simulink model "THEFINAL"  (R2020b)
settings: Solver=VariableStepAuto  StartTime=0.0  StopTime=60  RelTol=1e-3
values from neighbouring files (symbols this model uses):
  A_2 = zeros(3)    [Trial_Script.m]
  A_AD = horzcat(A_i, A_ii)    [Trial_Script.m]
  A_kal = [0 0 0 1 0 0 ... (first row only)    [Trial_Script.m]
  B_2 = I_inv    [Trial_Script.m]
  B_AD = horzcat(B_i, B_ii)    [Trial_Script.m]
  B_kal = [0 0 0 0 0 0 ... (first row only)    [Trial_Script.m]
  C_2 = eye(3)    [Trial_Script.m]
  C_AD = eye(6)    [Trial_Script.m]
  C_kal = eye(6)    [Trial_Script.m]
  D_2 = zeros(3)    [Trial_Script.m]
  D_AD = zeros(6)    [Trial_Script.m]
  D_kal = zeros(6)    [Trial_Script.m]
  f_prop = 100    [Trial_Script.m]
  Fb1_l = -100000    [Trial_Script.m]
  Fb1_u = 100000    [Trial_Script.m]
  Fb2_l = -100000    [Trial_Script.m]
  Fb2_u = 100000    [Trial_Script.m]
  Fb3_l = -100000    [Trial_Script.m]
  Fb3_u = 100000    [Trial_Script.m]
  Fb4_l = -100000    [Trial_Script.m]
  Fb4_u = 100000    [Trial_Script.m]
  Fc1_l = -30000    [Trial_Script.m]
  Fc1_u = 30000    [Trial_Script.m]
  Fc2_l = -30000    [Trial_Script.m]
  Fc2_u = 30000    [Trial_Script.m]
  Fc3_l = -30000    [Trial_Script.m]
  Fc3_u = 30000    [Trial_Script.m]
  Ft1_l = -100000    [Trial_Script.m]
  Ft1_u = 100000    [Trial_Script.m]
  Ft2_l = -100000    [Trial_Script.m]
  Ft2_u = 100000    [Trial_Script.m]
  Ft3_l = -100000    [Trial_Script.m]
  Ft3_u = 100000    [Trial_Script.m]
  Ft4_l = -100000    [Trial_Script.m]
  Ft4_u = 100000    [Trial_Script.m]
  g = 9.81    [Trial_Script.m]
  m = 645    [Trial_Script.m]    (also in testing_file.m = (abs(max(z)) + abs(min(z)))/(abs(max(y)) + abs(min(y))); wind_stuff.m = (abs(max(z)) + abs(min(z)))/(abs(max(y)) + abs(min(y))))
  r_0 = Tzy_Shard*[90; -125; 160]    [Trial_Script.m]
  rho = 1.225    [Trial_Script.m]
  T = 10.5    [Trial_Script.m]
  time_delay = 0.1    [Trial_Script.m]
  Tx_aero = [1 0 0 ... (first row only)    [Trial_Script.m]
  Tzy_Shard = [cos(pi/2) -sin(pi/2) 0; sin(pi/2) cos(pi/2) 0; 0 0 1]*[1 0 0 ... (first row only)    [Reading_Shard_Data.m]    (also in Trial_Script.m)
  Tzy_Shard_inv = inv(Tzy_Shard)    [Trial_Script.m]
  u_0 = a(1:d,1)    [Reading_Shard_Data.m]    (also in Trial_Script.m = a(1:d_shard,1); testing_file.m)
  u_1 = a(1:d,2)    [Reading_Shard_Data.m]    (also in Trial_Script.m = a(1:d_shard,2); testing_file.m)
  u_2 = a(1:d,3)    [Reading_Shard_Data.m]    (also in Trial_Script.m = a(1:d_shard,3); testing_file.m)
  v_0 = Tzy_Shard*V0_shard    [Trial_Script.m]
  w_0 = [0;0;0]    [Trial_Script.m]
  xdata = a(1:d_shard,4)    [Trial_Script.m]
  ydata = a(1:d_shard,5)    [Trial_Script.m]
  zdata = a(1:d_shard,6)    [Trial_Script.m]
  ZI_Cx = model_Cx(XI_Cx, YI_Cx)    [Trial_Script.m]
  ZI_Cy = model_Cy(XI_Cy, YI_Cy)    [Trial_Script.m]
  ZI_Cz = model_Cz(XI_Cz, YI_Cz)    [Trial_Script.m]
  ZI_p = model_p(XI_p, YI_p)    [Trial_Script.m]
  ZI_q = model_q(XI_q, YI_q)    [Trial_Script.m]
  ZI_r = model_r(XI_r, YI_r)    [Trial_Script.m]
undefined symbols (not defined in the file or in its folder): C_D, Continuous, S, Time
libraries: pid_lib x3, dspsigops x3, fuzblock x3, dspindex x3, ctrlSharedLib x2, simulink x1, mpclib x1, dspmathops x1, cstblocks x1
(part 1 of 2)
settings Model: Creator=Jonathan van Zyl  LastModifiedBy=Jonathan van Zyl

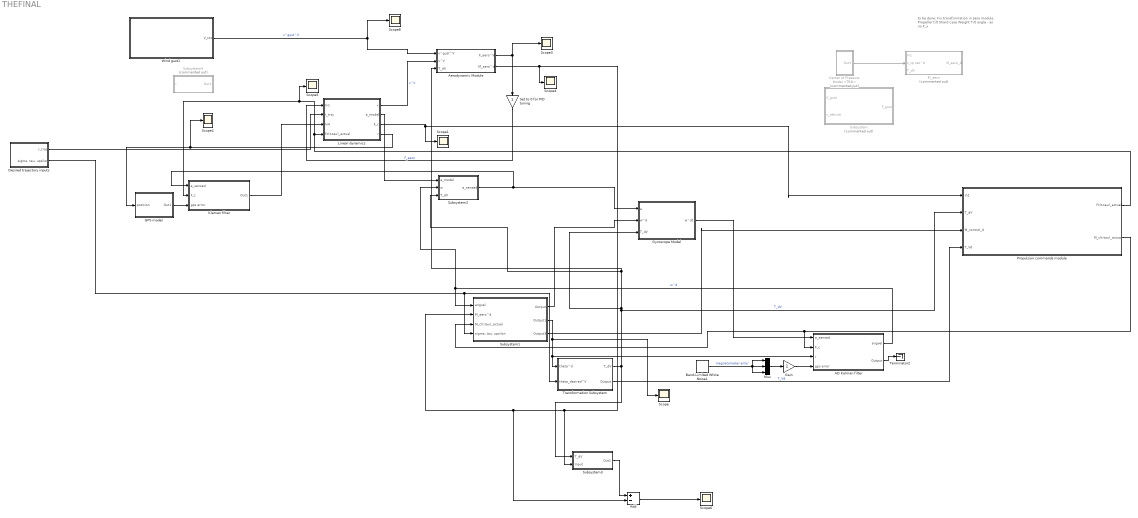
== system THEFINAL ==
  note: to be done:
      | Fix transformation in aero module
      | Propeller tilt
      | Shard case
      | Weight
      | Tilt angle - as no F_x
  AD Kalman filter : Subsystem
  Add : Sum  Inputs=+-
  Aerodynamic Module : Subsystem
  Band-Limited White Noise1 : simulink/Sources/Band-Limited White Noise  Cov=[0.000000001]  Ts=0.1  seed=[23341]
  Center of Pressure Model <TBD> : Subsystem  Commented=on
  Desired trajectory inputs : Subsystem
  GPS model : Subsystem
  Gain : Gain
  Gyroscope Model : Subsystem
  Klaman filter : Subsystem
  Linear dynamics : Subsystem
  M_aero : Subsystem  Commented=on
  Mux : Mux  Inputs=3
  Propulsion commands module : Subsystem
  Scope{,1..6,8} (8 alike) : Scope
  Set to 0 for PID tuning : Gain
  Subsystem : Subsystem  Commented=on
  Subsystem1 : Subsystem
  Subsystem2 : Subsystem
  Subsystem3 : Subsystem
  Subsystem4 : Subsystem  Commented=on
  Terminator2 : Terminator
  Transformation Subsystem : Subsystem
  Wind gust1 : Subsystem
  wires:
  Mux/1 -> Gain/1
  Subsystem3/1(Out1) -> Add/1
  Add/1 -> Scope6/1
  Propulsion commands module/1(Fc(t-tau)_actual) -> Scope5/1, Klaman filter/2(F_c), Linear dynamics/4(Fc(t-tau)_actual)
  Desired trajectory inputs/2("sigma, tau, upsilon") -> Transformation Subsystem/2(theta_desired^V), Subsystem1/4("sigma, tau, upsilon")
  Aerodynamic Module/1(F_aero^V) -> Set to 0 for PID tuning/1, Scope3/1
  Aerodynamic Module/2(M_aero^d) -> Scope4/1, Add/2, Subsystem1/2(M_aero^d), Subsystem3/2(Input)
  Wind gust1/1(V_tot) -> Aerodynamic Module/1(v^gust^V), Scope8/1  "v^gust^V"
  Linear dynamics/1(v) -> Aerodynamic Module/2(v^V)  "v^V"
  Gyroscope Model/1(w^d1) -> AD Kalman filter/1(a_sensed)
  Desired trajectory inputs/1(r_traj) -> Linear dynamics/2(r_traj)
  Propulsion commands module/2(M_c(t-tau)_actual) -> AD Kalman filter/2(F_c), Subsystem1/3(M_c(t-tau)_actual)
  Center of Pressure Model <TBD>/1(Out1) -> M_aero/2(x_cp vec^d)
  Transformation Subsystem/2(Output) -> Propulsion commands module/4(T_Vd)  "T_Vd"
  AD Kalman filter/2(Output) -> Terminator2/1
  Subsystem1/1(Output) -> Gyroscope Model/2(w^d)
  Subsystem1/2(Output1) -> Transformation Subsystem/1(theta^d), AD Kalman filter/3(r), Scope/1
  Subsystem1/3(Output3) -> Propulsion commands module/3(M_control_d)
  AD Kalman filter/1(angvel) -> Subsystem2/2(w), Subsystem1/1(angvel)  "w^d"
  Klaman filter/1(Out1) -> Linear dynamics/3(In4)
  Set to 0 for PID tuning/1 -> Linear dynamics/1(In1)  "F_aero"
  Band-Limited White Noise1/1 -> Mux/1, Mux/2, Mux/3  "magnetometer error"
  GPS model/1(Out1) -> Klaman filter/3(gps error)
  Subsystem2/1(a_sensed) -> Gyroscope Model/1(a), Klaman filter/1(a_sensed)
  Transformation Subsystem/1(T_dV) -> Subsystem3/1(T_dV), Aerodynamic Module/3(T_dV), Subsystem2/3(T_dV), Gyroscope Model/3(T_dV), Propulsion commands module/2(T_dV)  "T_dV"
  Linear dynamics/3(F_c) -> Propulsion commands module/1(In1), Scope1/1
  Gain/1 -> AD Kalman filter/4(gps error)
  Linear dynamics/4(r) -> GPS model/1(position), Scope2/1
  Linear dynamics/2(a_model) -> Subsystem2/1(a_model)

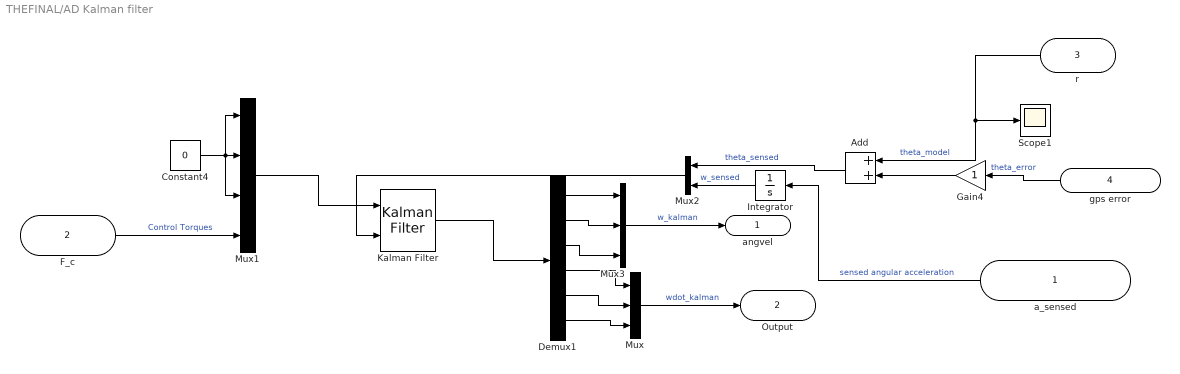
== system THEFINAL/AD Kalman filter ==
  a_sensed : Inport
  F_c : Inport  Port=2
  r : Inport  Port=3
  gps error : Inport  Port=4
  Add : Sum
  Constant4 : Constant  Value=0
  Demux1 : Demux  Outputs=6
  Gain4 : Gain
  Integrator : Integrator  InitialCondition=w_0
  Kalman Filter : ctrlSharedLib/Kalman Filter  TimeDomain=Continuous-Time  UseCurrentEstimator=on  ModelSource=Individual A, B, C, D matrices  ModelSourceVariable=ss(0.95,1,1,0,1)  A=A_AD  B=B_AD  C=C_AD  D=D_AD  NumberOfStates=1  NumberOfInputs=1  NumberOfOutputs=1  InitialEstimateSource=Dialog  X0=[0;0;0;0;0;0]  P0=10  UseK=off  UseGH=off  NumberOfProcessNoiseInputs=1  G=1  TimeInvariantG=on  H=0  TimeInvariantH=on  Q=0.05  TimeInvariantQ=on  R=1  TimeInvariantR=on  N=0  TimeInvariantN=on  AddInputPort=on  AddEnablePort=off  OutputEstimatedY=off  OutputP=off  Ts=-1
  Mux : Mux  Inputs=3
  Mux1 : Mux
  Mux2 : Mux  Inputs=2
  Mux3 : Mux  Inputs=3
  Scope1 : Scope
  angvel : Outport
  Output : Outport  Port=2
  wires:
  Demux1/5 -> Mux/2
  Mux2/1 -> Kalman Filter/2
  Constant4/1 -> Mux1/3, Mux1/1, Mux1/2
  gps error/1 -> Gain4/1  "theta_error"
  r/1 -> Scope1/1, Add/1  "theta_model"
  Demux1/4 -> Mux/1
  Demux1/2 -> Mux3/2
  Mux1/1 -> Kalman Filter/1
  F_c/1 -> Mux1/4  "Control Torques"
  Demux1/1 -> Mux3/1
  Kalman Filter/1 -> Demux1/1
  Demux1/6 -> Mux/3
  Gain4/1 -> Add/2
  Demux1/3 -> Mux3/3
  Integrator/1 -> Mux2/2  "w_sensed"
  Add/1 -> Mux2/1  "theta_sensed"
  Mux3/1 -> angvel/1  "w_kalman"
  a_sensed/1 -> Integrator/1  "sensed angular acceleration"
  Mux/1 -> Output/1  "wdot_kalman"

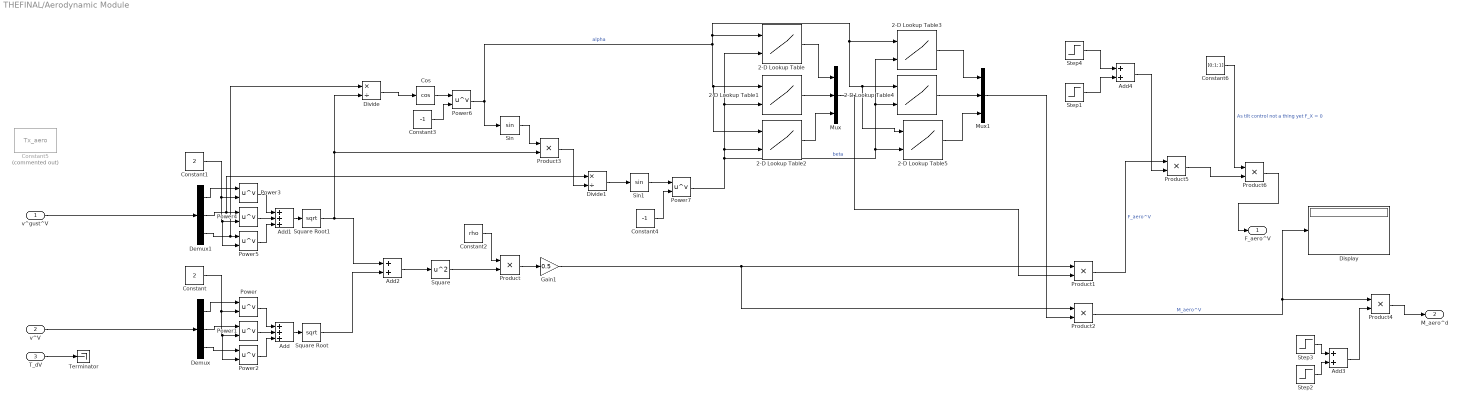
== system THEFINAL/Aerodynamic Module ==
  v^gust^V : Inport
  v^V : Inport  Port=2
  T_dV : Inport  Port=3
  2-D Lookup Table : Lookup_n-D  BreakpointsForDimension1=[-180:1:180]  BreakpointsForDimension2=[-180:1:180]  Table=ZI_Cx  InternalRulePriority=Speed  RndMeth=Simplest  InputSameDT=on
      settings: InputPortMap=u0,u1
  2-D Lookup Table1 : Lookup_n-D  BreakpointsForDimension1=[-180:1:180]  BreakpointsForDimension2=[-180:1:180]  Table=ZI_Cy  InternalRulePriority=Speed  RndMeth=Simplest  InputSameDT=on
      settings: InputPortMap=u0,u1
  2-D Lookup Table2 : Lookup_n-D  BreakpointsForDimension1=[-180:1:180]  BreakpointsForDimension2=[-180:1:180]  Table=ZI_Cz  InternalRulePriority=Speed  RndMeth=Simplest  InputSameDT=on
      settings: InputPortMap=u0,u1
  2-D Lookup Table3 : Lookup_n-D  BreakpointsForDimension1=[-180:1:180]  BreakpointsForDimension2=[-180:1:180]  Table=ZI_p  InternalRulePriority=Speed  RndMeth=Simplest  InputSameDT=on
      settings: InputPortMap=u0,u1
  2-D Lookup Table4 : Lookup_n-D  BreakpointsForDimension1=[-180:1:180]  BreakpointsForDimension2=[-180:1:180]  Table=ZI_q  InternalRulePriority=Speed  RndMeth=Simplest  InputSameDT=on
      settings: InputPortMap=u0,u1
  2-D Lookup Table5 : Lookup_n-D  BreakpointsForDimension1=[-180:1:180]  BreakpointsForDimension2=[-180:1:180]  Table=ZI_r  InternalRulePriority=Speed  RndMeth=Simplest  InputSameDT=on
      settings: InputPortMap=u0,u1
  Add : Sum  Inputs=+++
  Add1 : Sum  Inputs=+++
  Add2 : Sum
  Add3 : Sum
  Add4 : Sum
  Constant : Constant  Value=2
  Constant1 : Constant  Value=2
  Constant2 : Constant  Value=rho
  Constant3 : Constant  Value=-1
  Constant4 : Constant  Value=-1
  Constant5 : Constant  Commented=on  Value=Tx_aero
  Constant6 : Constant  Value=[0;1;1]
  Cos : Trigonometry  Operator=cos
  Demux : Demux  Outputs=3
  Demux1 : Demux  Outputs=3
  Display : Display
  Divide : Product  Inputs=*/
  Divide1 : Product  Inputs=*/
  Gain1 : Gain  Gain=0.5
  Mux : Mux  Inputs=3
  Mux1 : Mux  Inputs=3
  Power{,1..7} (8 alike) : Math  Operator=pow  SaturateOnIntegerOverflow=on
  Product{,1..6} (7 alike) : Product
  Sin : Trigonometry
  Sin1 : Trigonometry
  Square : Math  Operator=square  SaturateOnIntegerOverflow=on
  Square Root : Sqrt  SaturateOnIntegerOverflow=on
  Square Root1 : Sqrt  SaturateOnIntegerOverflow=on
  Step1 : Step  Time=0  SampleTime=0
  Step2 : Step  Time=0  SampleTime=0
  Step3 : Step  Time=10.5  After=-1  SampleTime=0
  Step4 : Step  Time=10.5  After=-1  SampleTime=0
  Terminator : Terminator
  F_aero^V : Outport
  M_aero^d : Outport  Port=2
  wires:
  Constant1/1 -> Power5/2, Power4/2, Power3/2
  Product1/1 -> Product5/1  "F_aero^V"
  Square Root/1 -> Add2/2
  Power6/1 -> Sin/1, 2-D Lookup Table/1, 2-D Lookup Table5/1, 2-D Lookup Table4/1, 2-D Lookup Table3/1, 2-D Lookup Table2/1, 2-D Lookup Table1/1  "alpha"
  Power1/1 -> Add/2
  2-D Lookup Table5/1 -> Mux1/3
  Constant/1 -> Power2/2, Power1/2, Power/2
  Divide/1 -> Cos/1
  Demux/1 -> Power/1
  Power5/1 -> Add1/3
  2-D Lookup Table/1 -> Mux/1
  Divide1/1 -> Sin1/1
  Demux1/1 -> Power3/1
  Add2/1 -> Square/1
  Product2/1 -> Display/1, Product4/1  "M_aero^V"
  Demux/3 -> Power2/1
  Constant4/1 -> Power7/2
  2-D Lookup Table4/1 -> Mux1/2
  Gain1/1 -> Product2/1, Product1/1
  Constant3/1 -> Power6/2
  Power7/1 -> 2-D Lookup Table/2, 2-D Lookup Table1/2, 2-D Lookup Table2/2, 2-D Lookup Table3/2, 2-D Lookup Table4/2, 2-D Lookup Table5/2  "beta"
  Cos/1 -> Power6/1
  Demux1/3 -> Divide/1, Power5/1
  Product/1 -> Gain1/1
  Sin1/1 -> Power7/1
  Power2/1 -> Add/3
  Sin/1 -> Product3/1
  Mux1/1 -> Product2/2
  Demux1/2 -> Divide1/1, Power4/1
  Power4/1 -> Add1/2
  Add/1 -> Square Root/1
  Power/1 -> Add/1
  Square Root1/1 -> Product3/2, Divide/2, Add2/1
  2-D Lookup Table3/1 -> Mux1/1
  2-D Lookup Table1/1 -> Mux/2
  Power3/1 -> Add1/1
  Mux/1 -> Product1/2
  Product3/1 -> Divide1/2
  2-D Lookup Table2/1 -> Mux/3
  Add1/1 -> Square Root1/1
  Constant2/1 -> Product/1
  Demux/2 -> Power1/1
  Add3/1 -> Product4/2
  Step3/1 -> Add3/1
  Step2/1 -> Add3/2
  Product4/1 -> M_aero^d/1
  Step4/1 -> Add4/1
  Step1/1 -> Add4/2
  Square/1 -> Product/2
  Constant6/1 -> Product6/1  "As tilt control not a thing yet F_X = 0"
  Product6/1 -> F_aero^V/1
  T_dV/1 -> Terminator/1
  v^V/1 -> Demux/1
  Product5/1 -> Product6/2
  Add4/1 -> Product5/2
  v^gust^V/1 -> Demux1/1

== system THEFINAL/Center of Pressure Model <TBD> ==
  Constant1 : Constant  Value=[0.1;0.2; 0.05]
  Out1 : Outport
  wires:
  Constant1/1 -> Out1/1  "x_cp"

== system THEFINAL/Desired trajectory inputs ==
  Constant : Constant  Value=Tzy_Shard
  Constant1 : Constant  Value=[90; 174; 240]
  Constant2 : Constant  Value=[0;1;1]
  Constant3 : Constant  Value=[0;10*pi/180;0]
  Matrix Multiply : Product  Multiplication=Matrix(*)
  Product : Product
  r_traj : Outport
  "sigma, tau, upsilon" : Outport  Port=2
  wires:
  Product/1 -> r_traj/1  "r_traj"
  Constant3/1 -> "sigma, tau, upsilon"/1  "sigma, tau, upsilon"
  Constant/1 -> Matrix Multiply/1
  Constant1/1 -> Matrix Multiply/2
  Constant2/1 -> Product/1
  Matrix Multiply/1 -> Product/2  "r_traj"

== system THEFINAL/GPS model ==
  position : Inport
  GPS Model : MATLAB Function  TreatAsAtomicUnit=on
  Transpose : Math  Operator=transpose  SaturateOnIntegerOverflow=on
  Out1 : Outport
  wires:
  GPS Model/1(newposition) -> Transpose/1  "gps error"
  position/1 -> GPS Model/1(position)
  Transpose/1 -> Out1/1  "r_sensed"

== system THEFINAL/Gyroscope Model ==
  a : Inport
  w^d : Inport  Port=2
  T_dV : Inport  Port=3
  Demux : Demux  Outputs=3
  MATLAB Function : MATLAB Function  TreatAsAtomicUnit=on
  Terminator : Terminator
  Transpose : Math  Operator=transpose  SaturateOnIntegerOverflow=on
  Transpose2 : Math  Operator=transpose  SaturateOnIntegerOverflow=on
  w^d1 : Outport
  wires:
  T_dV/1 -> Terminator/1
  Transpose2/1 -> w^d1/1
  MATLAB Function/1(gyroData) -> Transpose2/1
  a/1 -> Transpose/1
  Transpose/1 -> MATLAB Function/4(acc)
  w^d/1 -> Demux/1
  Demux/1 -> MATLAB Function/1(xvel)
  Demux/2 -> MATLAB Function/2(yvel)
  Demux/3 -> MATLAB Function/3(zvel)

== system THEFINAL/Klaman filter ==
  a_sensed : Inport
  F_c : Inport  Port=2
  gps error : Inport  Port=3
  Constant4 : Constant  Value=0
  Demux1 : Demux  Outputs=6
  Integrator : Integrator  InitialCondition=v_0
  Kalman Filter : ctrlSharedLib/Kalman Filter  TimeDomain=Continuous-Time  UseCurrentEstimator=on  ModelSource=Individual A, B, C, D matrices  ModelSourceVariable=ss(0.95,1,1,0,1)  A=A_kal  B=B_kal  C=C_kal  D=D_kal  NumberOfStates=1  NumberOfInputs=1  NumberOfOutputs=1  InitialEstimateSource=Dialog  X0=[0;0;0;0;0;0]  P0=10  UseK=off  UseGH=off  NumberOfProcessNoiseInputs=1  G=1  TimeInvariantG=on  H=0  TimeInvariantH=on  Q=0.05  TimeInvariantQ=on  R=1  TimeInvariantR=on  N=0  TimeInvariantN=on  AddInputPort=on  AddEnablePort=off  OutputEstimatedY=off  OutputP=off  Ts=-1
  Mux1 : Mux
  Mux2 : Mux  Inputs=2
  Mux3 : Mux  Inputs=3
  Terminator : Terminator
  Terminator1 : Terminator
  Terminator2 : Terminator
  Out1 : Outport
  wires:
  Demux1/5 -> Terminator1/1
  Mux2/1 -> Kalman Filter/2
  Constant4/1 -> Mux1/3, Mux1/1, Mux1/2
  Demux1/4 -> Terminator/1
  Demux1/2 -> Mux3/2
  Mux1/1 -> Kalman Filter/1
  F_c/1 -> Mux1/4  "Control Force"
  Demux1/1 -> Mux3/1
  Kalman Filter/1 -> Demux1/1
  Demux1/6 -> Terminator2/1
  Demux1/3 -> Mux3/3
  Integrator/1 -> Mux2/2  "v_sensed"
  gps error/1 -> Mux2/1  "r_sensed"
  Mux3/1 -> Out1/1  "r_kalman"
  a_sensed/1 -> Integrator/1  "sensed acceleration"

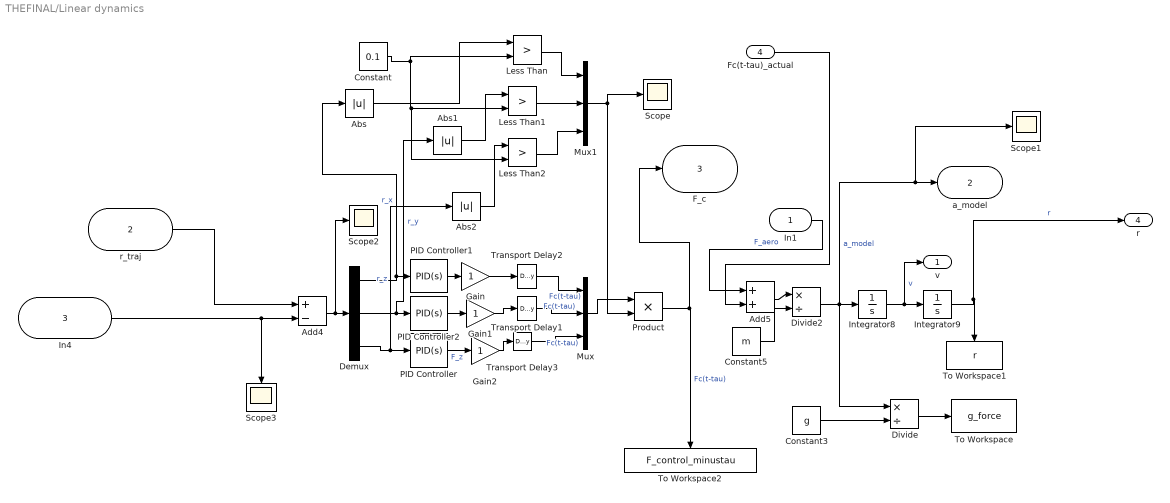
== system THEFINAL/Linear dynamics ==
  In1 : Inport
  r_traj : Inport  Port=2
  In4 : Inport  Port=3
  Fc(t-tau)_actual : Inport  Port=4
  Abs : Abs
  Abs1 : Abs
  Abs2 : Abs
  Add4 : Sum  Inputs=+-
  Add5 : Sum
  Constant : Constant  Value=0.1
  Constant3 : Constant  Value=g
  Constant5 : Constant  Value=m
  Demux : Demux  Outputs=3
  Divide : Product  Inputs=*/
  Divide2 : Product  Inputs=*/
  Gain : Gain
  Gain1 : Gain
  Gain2 : Gain
  Integrator8 : Integrator  InitialCondition=v_0
  Integrator9 : Integrator  InitialCondition=r_0
  Less Than : RelationalOperator  Operator=>  OutDataTypeStr=boolean  RndMeth=Simplest
  Less Than1 : RelationalOperator  Operator=>  OutDataTypeStr=boolean  RndMeth=Simplest
  Less Than2 : RelationalOperator  Operator=>  OutDataTypeStr=boolean  RndMeth=Simplest
  Mux : Mux  Inputs=3
  Mux1 : Mux  Inputs=3
  PID Controller : pid_lib/PID Controller  Controller=PID  Form=Parallel  TimeDomain=Continuous-time  UseExternalTs=off  SampleTime=-1  IntegratorMethod=Forward Euler  FilterMethod=Forward Euler  ControllerParametersSource=internal  P=9009.63914576468  I=3464.3602040453  D=5659.73322598295  UseFilter=on  N=27.0214258529072  TunerSelectOption=Transfer Function Based (PID Tuner App)  InitialConditionSource=internal  InitialConditionForIntegrator=0  InitialConditionForFilter=0  DifferentiatorICPrevScaledInput=0  ExternalReset=none  TrackingMode=off  Kt=1  LimitOutput=off  SatLimitsSource=internal  UpperSaturationLimit=inf  LowerSaturationLimit=-inf  LinearizeAsGain=on  AntiWindupMode=none  Kb=1  POutMin=[]  POutMax=[]  IOutMin=[]  IOutMax=[]  DOutMin=[]  DOutMax=[]  NOutMin=[]  NOutMax=[]  SumOutMin=[]  SumOutMax=[]  SaturationOutMin=[]  SaturationOutMax=[]  PParamMin=[]  PParamMax=[]  IParamMin=[]  IParamMax=[]  DParamMin=[]  DParamMax=[]  NParamMin=[]  NParamMax=[]  KbParamMin=[]  KbParamMax=[]  KtParamMin=[]  KtParamMax=[]  KbOutMin=[]  KbOutMax=[]  KtOutMin=[]  KtOutMax=[]  IntegratorOutMin=[]  IntegratorOutMax=[]  FilterOutMin=[]  FilterOutMax=[]  SumI1OutMin=[]  SumI1OutMax=[]  SumI2OutMin=[]  SumI2OutMax=[]  SumI3OutMin=[]  SumI3OutMax=[]  SumI4OutMin=[]  SumI4OutMax=[]  SumDOutMin=[]  SumDOutMax=[]  DifferentiatorOutMin=[]  DifferentiatorOutMax=[]  FilterDiffOutCoefMin=[]  FilterDiffOutCoefMax=[]  ReciprocalOutMin=[]  ReciprocalOutMax=[]  SumDenOutMin=[]  SumDenOutMax=[]  SumNumOutMin=[]  SumNumOutMax=[]  DivideOutMin=[]  DivideOutMax=[]  UdiffTsProdOutMin=[]  UdiffTsProdOutMax=[]  NTsProdOutMin=[]  NTsProdOutMax=[]  UintegralTsProdOutMin=[]  UintegralTsProdOutMax=[]  UngainTsProdOutMin=[]  UngainTsProdOutMax=[]  IntegratorContinuousStateAttributes=''  IntegratorStateMustResolveToSignalObject=off  IntegratorRTWStateStorageClass=Auto  FilterContinuousStateAttributes=''  FilterStateMustResolveToSignalObject=off  FilterRTWStateStorageClass=Auto  ParallelPVariant=InternalParameters  IdealPVariant=Disabled  IVariant=InternalParameters  DVariant=InternalParameters  IntegratorVariant=Continuous  SatVariant=Disabled  AWVariant=Passthrough  PCopyVariant=Disabled  TRVariant=Disabled  FdbkBlocksVariant=Forward  IdealPFdbkVariant=Disabled  SatFdbkVariant=Disabled  DerivativeFilterVariant=ContFilter  NVariant=InternalParameters  NCopyVariant=Disabled  FilterICVariant=InternalICsFilter  IntegratorICVariant=InternalICs  ExternalResetVariant=Disabled  TRSumVariant=Passthrough  SumFdbkVariant=Disabled  SumVariant=Sum_PID  TsampFilterVariant=InternalTs  TsampNgainVariant=Passthrough  TsampIntegralVariant=Passthrough  ExternalSaturationOutDataTypeStr=Inherit: Same as second input
  PID Controller1 : pid_lib/PID Controller  Controller=PID  Form=Parallel  TimeDomain=Continuous-time  UseExternalTs=off  SampleTime=-1  IntegratorMethod=Forward Euler  FilterMethod=Forward Euler  ControllerParametersSource=internal  P=9009.63914576468  I=3464.36020404063  D=5659.73322596604  UseFilter=on  N=27.0214258528983  TunerSelectOption=Transfer Function Based (PID Tuner App)  InitialConditionSource=internal  InitialConditionForIntegrator=0  InitialConditionForFilter=0  DifferentiatorICPrevScaledInput=0  ExternalReset=none  TrackingMode=off  Kt=1  LimitOutput=off  SatLimitsSource=internal  UpperSaturationLimit=inf  LowerSaturationLimit=-inf  LinearizeAsGain=on  AntiWindupMode=none  Kb=1  POutMin=[]  POutMax=[]  IOutMin=[]  IOutMax=[]  DOutMin=[]  DOutMax=[]  NOutMin=[]  NOutMax=[]  SumOutMin=[]  SumOutMax=[]  SaturationOutMin=[]  SaturationOutMax=[]  PParamMin=[]  PParamMax=[]  IParamMin=[]  IParamMax=[]  DParamMin=[]  DParamMax=[]  NParamMin=[]  NParamMax=[]  KbParamMin=[]  KbParamMax=[]  KtParamMin=[]  KtParamMax=[]  KbOutMin=[]  KbOutMax=[]  KtOutMin=[]  KtOutMax=[]  IntegratorOutMin=[]  IntegratorOutMax=[]  FilterOutMin=[]  FilterOutMax=[]  SumI1OutMin=[]  SumI1OutMax=[]  SumI2OutMin=[]  SumI2OutMax=[]  SumI3OutMin=[]  SumI3OutMax=[]  SumI4OutMin=[]  SumI4OutMax=[]  SumDOutMin=[]  SumDOutMax=[]  DifferentiatorOutMin=[]  DifferentiatorOutMax=[]  FilterDiffOutCoefMin=[]  FilterDiffOutCoefMax=[]  ReciprocalOutMin=[]  ReciprocalOutMax=[]  SumDenOutMin=[]  SumDenOutMax=[]  SumNumOutMin=[]  SumNumOutMax=[]  DivideOutMin=[]  DivideOutMax=[]  UdiffTsProdOutMin=[]  UdiffTsProdOutMax=[]  NTsProdOutMin=[]  NTsProdOutMax=[]  UintegralTsProdOutMin=[]  UintegralTsProdOutMax=[]  UngainTsProdOutMin=[]  UngainTsProdOutMax=[]  IntegratorContinuousStateAttributes=''  IntegratorStateMustResolveToSignalObject=off  IntegratorRTWStateStorageClass=Auto  FilterContinuousStateAttributes=''  FilterStateMustResolveToSignalObject=off  FilterRTWStateStorageClass=Auto  ParallelPVariant=InternalParameters  IdealPVariant=Disabled  IVariant=InternalParameters  DVariant=InternalParameters  IntegratorVariant=Continuous  SatVariant=Disabled  AWVariant=Passthrough  PCopyVariant=Disabled  TRVariant=Disabled  FdbkBlocksVariant=Forward  IdealPFdbkVariant=Disabled  SatFdbkVariant=Disabled  DerivativeFilterVariant=ContFilter  NVariant=InternalParameters  NCopyVariant=Disabled  FilterICVariant=InternalICsFilter  IntegratorICVariant=InternalICs  ExternalResetVariant=Disabled  TRSumVariant=Passthrough  SumFdbkVariant=Disabled  SumVariant=Sum_PID  TsampFilterVariant=InternalTs  TsampNgainVariant=Passthrough  TsampIntegralVariant=Passthrough  ExternalSaturationOutDataTypeStr=Inherit: Same as second input
  PID Controller2 : pid_lib/PID Controller  Controller=PID  Form=Parallel  TimeDomain=Continuous-time  UseExternalTs=off  SampleTime=-1  IntegratorMethod=Forward Euler  FilterMethod=Forward Euler  ControllerParametersSource=internal  P=9009.63914576468  I=3464.36020397681  D=5659.73322587286  UseFilter=on  N=27.0214258527793  TunerSelectOption=Transfer Function Based (PID Tuner App)  InitialConditionSource=internal  InitialConditionForIntegrator=0  InitialConditionForFilter=0  DifferentiatorICPrevScaledInput=0  ExternalReset=none  TrackingMode=off  Kt=1  LimitOutput=off  SatLimitsSource=internal  UpperSaturationLimit=inf  LowerSaturationLimit=-inf  LinearizeAsGain=on  AntiWindupMode=none  Kb=1  POutMin=[]  POutMax=[]  IOutMin=[]  IOutMax=[]  DOutMin=[]  DOutMax=[]  NOutMin=[]  NOutMax=[]  SumOutMin=[]  SumOutMax=[]  SaturationOutMin=[]  SaturationOutMax=[]  PParamMin=[]  PParamMax=[]  IParamMin=[]  IParamMax=[]  DParamMin=[]  DParamMax=[]  NParamMin=[]  NParamMax=[]  KbParamMin=[]  KbParamMax=[]  KtParamMin=[]  KtParamMax=[]  KbOutMin=[]  KbOutMax=[]  KtOutMin=[]  KtOutMax=[]  IntegratorOutMin=[]  IntegratorOutMax=[]  FilterOutMin=[]  FilterOutMax=[]  SumI1OutMin=[]  SumI1OutMax=[]  SumI2OutMin=[]  SumI2OutMax=[]  SumI3OutMin=[]  SumI3OutMax=[]  SumI4OutMin=[]  SumI4OutMax=[]  SumDOutMin=[]  SumDOutMax=[]  DifferentiatorOutMin=[]  DifferentiatorOutMax=[]  FilterDiffOutCoefMin=[]  FilterDiffOutCoefMax=[]  ReciprocalOutMin=[]  ReciprocalOutMax=[]  SumDenOutMin=[]  SumDenOutMax=[]  SumNumOutMin=[]  SumNumOutMax=[]  DivideOutMin=[]  DivideOutMax=[]  UdiffTsProdOutMin=[]  UdiffTsProdOutMax=[]  NTsProdOutMin=[]  NTsProdOutMax=[]  UintegralTsProdOutMin=[]  UintegralTsProdOutMax=[]  UngainTsProdOutMin=[]  UngainTsProdOutMax=[]  IntegratorContinuousStateAttributes=''  IntegratorStateMustResolveToSignalObject=off  IntegratorRTWStateStorageClass=Auto  FilterContinuousStateAttributes=''  FilterStateMustResolveToSignalObject=off  FilterRTWStateStorageClass=Auto  ParallelPVariant=InternalParameters  IdealPVariant=Disabled  IVariant=InternalParameters  DVariant=InternalParameters  IntegratorVariant=Continuous  SatVariant=Disabled  AWVariant=Passthrough  PCopyVariant=Disabled  TRVariant=Disabled  FdbkBlocksVariant=Forward  IdealPFdbkVariant=Disabled  SatFdbkVariant=Disabled  DerivativeFilterVariant=ContFilter  NVariant=InternalParameters  NCopyVariant=Disabled  FilterICVariant=InternalICsFilter  IntegratorICVariant=InternalICs  ExternalResetVariant=Disabled  TRSumVariant=Passthrough  SumFdbkVariant=Disabled  SumVariant=Sum_PID  TsampFilterVariant=InternalTs  TsampNgainVariant=Passthrough  TsampIntegralVariant=Passthrough  ExternalSaturationOutDataTypeStr=Inherit: Same as second input
  Product : Product
  Scope{,1..3} (4 alike) : Scope
  To Workspace : ToWorkspace  VariableName=g_force  SaveFormat=Timeseries  SampleTime=-1
      settings: Save2DSignal=2-D array (concatenate along first dimension)
  To Workspace1 : ToWorkspace  VariableName=r  SaveFormat=Timeseries  SampleTime=-1
  To Workspace2 : ToWorkspace  VariableName=F_control_minustau  SaveFormat=Timeseries  SampleTime=-1
  Transport Delay1 : TransportDelay  DelayTime=time_delay  TransDelayFeedthrough=on
  Transport Delay2 : TransportDelay  DelayTime=time_delay  TransDelayFeedthrough=on
  Transport Delay3 : TransportDelay  DelayTime=time_delay  TransDelayFeedthrough=on
  v : Outport
  a_model : Outport  Port=2
  F_c : Outport  Port=3
  r : Outport  Port=4
  wires:
  Divide2/1 -> Divide/1, Scope1/1, a_model/1, Integrator8/1  "a_model"
  In4/1 -> Add4/2, Scope3/1
  Divide/1 -> To Workspace/1
  r_traj/1 -> Add4/1
  PID Controller2/1 -> Gain1/1
  Add5/1 -> Divide2/1
  Constant5/1 -> Divide2/2
  Demux/1 -> Abs/1, PID Controller1/1  "r_x"
  PID Controller/1 -> Gain2/1  "F_z"
  Gain1/1 -> Transport Delay1/1
  Add4/1 -> Scope2/1, Demux/1
  Integrator9/1 -> r/1, To Workspace1/1  "r"
  Demux/2 -> Abs1/1, PID Controller2/1  "r_y"
  Product/1 -> F_c/1, To Workspace2/1  "Fc(t-tau)"
  PID Controller1/1 -> Gain/1
  Constant3/1 -> Divide/2
  Gain/1 -> Transport Delay2/1
  Demux/3 -> Abs2/1, PID Controller/1  "r_z"
  Gain2/1 -> Transport Delay3/1
  Integrator8/1 -> Integrator9/1, v/1  "v"
  In1/1 -> Add5/1  "F_aero"
  Transport Delay2/1 -> Mux/1  "Fc(t-tau)"
  Transport Delay1/1 -> Mux/2  "Fc(t-tau)"
  Transport Delay3/1 -> Mux/3  "Fc(t-tau)"
  Constant/1 -> Less Than2/2, Less Than1/2, Less Than/2
  Less Than1/1 -> Mux1/2
  Less Than/1 -> Mux1/1
  Less Than2/1 -> Mux1/3
  Mux/1 -> Product/1
  Abs/1 -> Less Than/1
  Abs1/1 -> Less Than1/1
  Abs2/1 -> Less Than2/1
  Fc(t-tau)_actual/1 -> Add5/2
  Mux1/1 -> Product/2, Scope/1

== system THEFINAL/M_aero ==
  In1 : Inport
  x_cp vec^d : Inport  Port=2
  T_dV : Inport  Port=3
  Matrix Multiply : Product  Multiplication=Matrix(*)
  Matrix Multiply1 : Product
  M_aero_d : Outport
  wires:
  Matrix Multiply/1 -> Matrix Multiply1/2  "F_dis^d"
  x_cp vec^d/1 -> Matrix Multiply1/1  "x_cp"
  T_dV/1 -> Matrix Multiply/1
  In1/1 -> Matrix Multiply/2  "F_gust"
  Matrix Multiply1/1 -> M_aero_d/1  "M_aero_d"

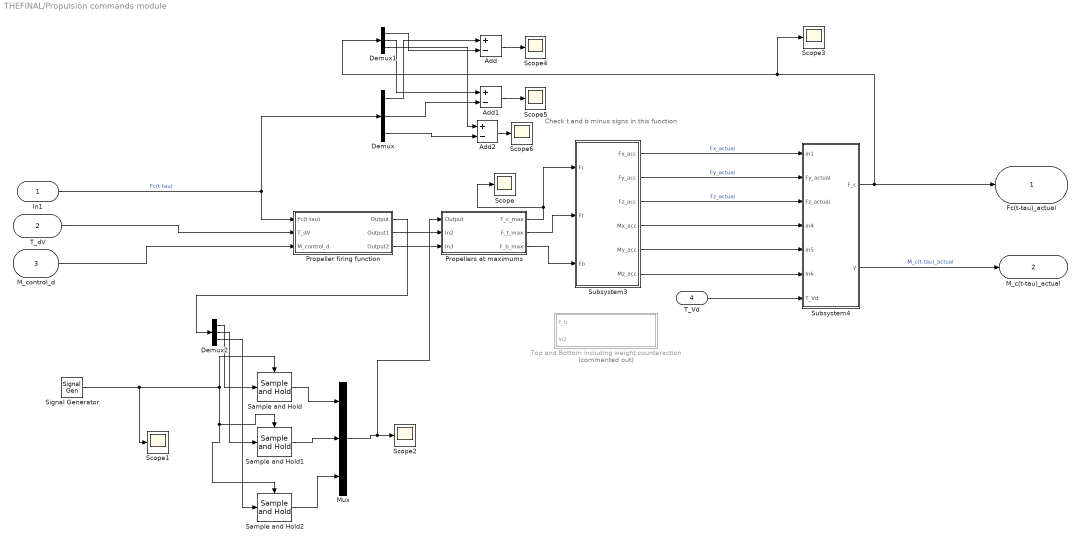
== system THEFINAL/Propulsion commands module ==
  note: Check t and b minus signs in this function
  In1 : Inport
  T_dV : Inport  Port=2
  M_control_d : Inport  Port=3
  T_Vd : Inport  Port=4
  Add : Sum  Inputs=+-
  Add1 : Sum  Inputs=+-
  Add2 : Sum  Inputs=+-
  Demux : Demux  Outputs=3
  Demux1 : Demux  Outputs=3
  Demux2 : Demux  Outputs=3
  Mux : Mux  Inputs=3
  Propeller firing function : Subsystem
  Propellers at maximums : Subsystem
  Sample and Hold : dspsigops/Sample and Hold  trig=Either edge  initCond=0  latchinput=off
  Sample and Hold1 : dspsigops/Sample and Hold  trig=Either edge  initCond=0  latchinput=off
  Sample and Hold2 : dspsigops/Sample and Hold  trig=Either edge  initCond=0  latchinput=off
  Scope{,1..6} (7 alike) : Scope
  Signal Generator : SignalGenerator  WaveForm=square  Frequency=f_prop  Units=rad/sec
  Subsystem3 : Subsystem
  Subsystem4 : Subsystem
  Top and Bottom including weight counteraction : Subsystem  Commented=on
  Fc(t-tau)_actual : Outport
  M_c(t-tau)_actual : Outport  Port=2
  wires:
  Subsystem3/2(Fy_acc) -> Subsystem4/2(Fy_actual)  "Fy_actual"
  Subsystem4/1(F_c) -> Fc(t-tau)_actual/1, Scope3/1, Demux1/1
  Demux1/3 -> Add2/1
  Subsystem3/3(Fz_acc) -> Subsystem4/3(Fz_actual)  "Fz_actual"
  Demux/2 -> Add1/2
  T_dV/1 -> Propeller firing function/2(T_dV)
  Subsystem3/1(Fx_acc) -> Subsystem4/1(In1)  "Fx_actual"
  Demux1/2 -> Add1/1
  Propeller firing function/1(Output) -> Demux2/1
  Propellers at maximums/2(F_t_max) -> Subsystem3/2(Ft)
  Demux1/1 -> Add/2
  Propeller firing function/2(Output1) -> Propellers at maximums/2(In2)
  Subsystem3/5(My_acc) -> Subsystem4/5(In5)
  Subsystem3/6(Mz_acc) -> Subsystem4/6(In6)
  Propellers at maximums/3(F_b_max) -> Subsystem3/3(Fb)
  Demux/3 -> Add2/2
  Subsystem4/2(y) -> M_c(t-tau)_actual/1  "M_c(t-tau)_actual"
  Propeller firing function/3(Output2) -> Propellers at maximums/3(In3)
  In1/1 -> Demux/1, Propeller firing function/1(Fc(t-tau))  "Fc(t-tau)"
  T_Vd/1 -> Subsystem4/7(T_Vd)
  Subsystem3/4(Mx_acc) -> Subsystem4/4(In4)
  Add1/1 -> Scope5/1
  Propellers at maximums/1(F_c_max) -> Scope/1, Subsystem3/1(Fc)
  Add2/1 -> Scope6/1
  Demux/1 -> Add/1
  Add/1 -> Scope4/1
  M_control_d/1 -> Propeller firing function/3(M_control_d)
  Sample and Hold/1 -> Mux/1
  Signal Generator/1 -> Scope1/1, Sample and Hold/Trigger, Sample and Hold2/Trigger, Sample and Hold1/Trigger
  Demux2/1 -> Sample and Hold/1
  Demux2/2 -> Sample and Hold1/1
  Sample and Hold1/1 -> Mux/2
  Sample and Hold2/1 -> Mux/3
  Mux/1 -> Propellers at maximums/1(Output), Scope2/1
  Demux2/3 -> Sample and Hold2/1

== system THEFINAL/Subsystem ==
  V_gust : Inport
  v_vehicle : Inport  Port=2
  Add2 : Sum
  Add3 : Sum
  Drag1 : Subsystem
  Product : Product
  Scope : Scope
  Step2 : Step  Time=0  SampleTime=0
  Step3 : Step  Time=10.5  After=-1  SampleTime=0
  To Workspace : ToWorkspace  VariableName=v_sumsq  SampleTime=-1
  To Workspace1 : ToWorkspace  VariableName=step  SaveFormat=Timeseries  SampleTime=-1
  To Workspace2 : ToWorkspace  VariableName=vtotal  SaveFormat=Timeseries  SampleTime=-1
  To Workspace3 : ToWorkspace  VariableName=F_gust  SaveFormat=Timeseries  SampleTime=-1
  To Workspace4 : ToWorkspace  VariableName=v_gust  SaveFormat=Timeseries  SampleTime=-1
  F_gust : Outport
  wires:
  Product/1 -> F_gust/1, To Workspace3/1, Scope/1  "F_gust"
  Step3/1 -> Add2/1
  V_gust/1 -> To Workspace4/1, Add3/1
  Drag1/1(Out1) -> To Workspace/1
  Add3/1 -> Drag1/1(In1), To Workspace2/1
  Add2/1 -> To Workspace1/1, Product/2
  Step2/1 -> Add2/2
  v_vehicle/1 -> Add3/2
  Drag1/2(drag) -> Product/1

== system THEFINAL/Subsystem1 ==
  angvel : Inport
  M_aero^d : Inport  Port=2
  M_c(t-tau)_actual : Inport  Port=3
  "sigma, tau, upsilon" : Inport  Port=4
  Subsystem : Subsystem
  Output : Outport
  Output1 : Outport  Port=2
  Output3 : Outport  Port=3
  wires:
  M_aero^d/1 -> Subsystem/1(M_aero^d)  "M_aero^d"
  "sigma, tau, upsilon"/1 -> Subsystem/2(Input)  "sigma, tau upsilon"
  Subsystem/1(Output) -> Output1/1  "theta^d"
  Subsystem/2(Output1) -> Output3/1
  Subsystem/3(Out1) -> Output/1
  angvel/1 -> Subsystem/3(angvel)  "angelvel"
  M_c(t-tau)_actual/1 -> Subsystem/4(M_c(t-tau)_actual)

== system THEFINAL/Subsystem2 ==
  a_model : Inport
  w : Inport  Port=2
  T_dV : Inport  Port=3
  Display : Display
  Display1 : Display
  MATLAB Function : MATLAB Function  Commented=on  TreatAsAtomicUnit=on
  Terminator : Terminator
  Terminator3 : Terminator
  Transpose : Math  Operator=transpose  SaturateOnIntegerOverflow=on
  Transpose1 : Math  Operator=transpose  SaturateOnIntegerOverflow=on
  Transpose2 : Math  Operator=transpose  SaturateOnIntegerOverflow=on
  a_sensed : Outport
  wires:
  T_dV/1 -> Terminator3/1
  a_model/1 -> Transpose1/1
  Transpose2/1 -> a_sensed/1  "a_sensed"
  w/1 -> Transpose/1
  Transpose/1 -> Terminator/1
  Transpose1/1 -> Display1/1, Transpose2/1, Display/1  "a_sensed"

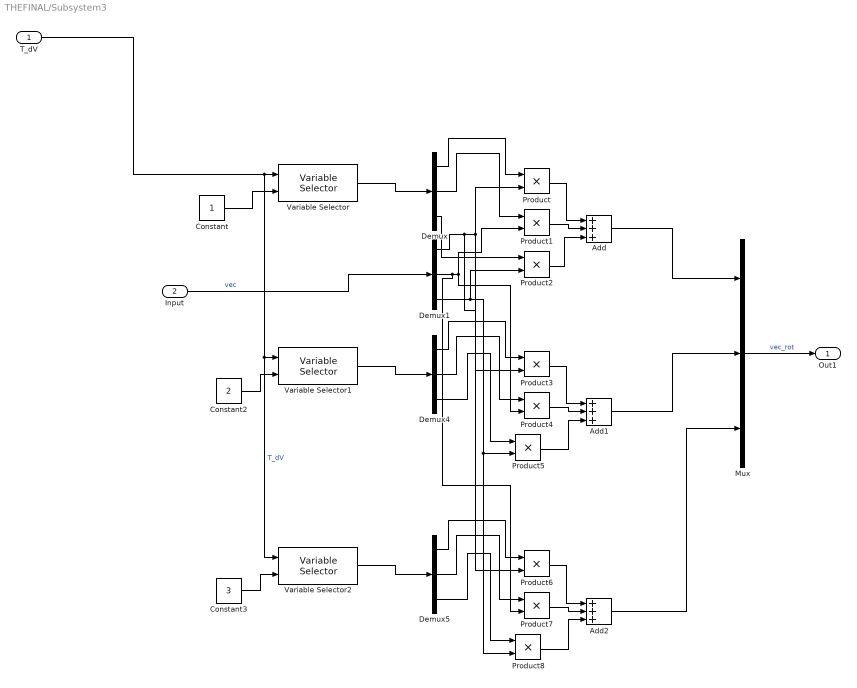
== system THEFINAL/Subsystem3 ==
  T_dV : Inport
  Input : Inport  Port=2
  Add : Sum  Inputs=+++
  Add1 : Sum  Inputs=+++
  Add2 : Sum  Inputs=+++
  Constant : Constant
  Constant2 : Constant  Value=2
  Constant3 : Constant  Value=3
  Demux{,1,4..5} (4 alike) : Demux  Outputs=3
  Mux : Mux  Inputs=3
  Product{,1..8} (9 alike) : Product
  Variable Selector : dspindex/Variable Selector  NumInputs=1  rowsOrCols=Columns  IdxMode=Variable  Elements=[1 3]  ZerOneIdxMode=One-based  errmode=Clip Index  FillMode=on  FillValues=0
  Variable Selector1 : dspindex/Variable Selector  NumInputs=1  rowsOrCols=Columns  IdxMode=Variable  Elements=[1 3]  ZerOneIdxMode=One-based  errmode=Clip Index  FillMode=on  FillValues=0
  Variable Selector2 : dspindex/Variable Selector  NumInputs=1  rowsOrCols=Columns  IdxMode=Variable  Elements=[1 3]  ZerOneIdxMode=One-based  errmode=Clip Index  FillMode=on  FillValues=0
  Out1 : Outport
  wires:
  Variable Selector/1 -> Demux/1
  Add2/1 -> Mux/3
  Demux/1 -> Product/1
  Product3/1 -> Add1/1
  Variable Selector1/1 -> Demux4/1
  Product4/1 -> Add1/2
  Demux4/2 -> Product4/1
  Demux/2 -> Product1/1
  Constant2/1 -> Variable Selector1/2
  Constant/1 -> Variable Selector/2
  Mux/1 -> Out1/1  "vec_rot"
  Add/1 -> Mux/1
  Product5/1 -> Add1/3
  Demux1/2 -> Product7/2, Product1/2, Product4/2
  Product/1 -> Add/1
  Demux5/2 -> Product7/1
  Product8/1 -> Add2/3
  Demux5/3 -> Product8/1
  Product7/1 -> Add2/2
  Demux5/1 -> Product6/1
  Product6/1 -> Add2/1
  Constant3/1 -> Variable Selector2/2
  Demux/3 -> Product2/1
  Variable Selector2/1 -> Demux5/1
  Demux1/3 -> Product8/2, Product5/2, Product2/2
  Product2/1 -> Add/3
  Add1/1 -> Mux/2
  Product1/1 -> Add/2
  Demux4/1 -> Product3/1
  Demux4/3 -> Product5/1
  T_dV/1 -> Variable Selector2/1, Variable Selector1/1, Variable Selector/1  "T_dV"
  Demux1/1 -> Product6/2, Product/2, Product3/2
  Input/1 -> Demux1/1  "vec"

== system THEFINAL/Subsystem4 ==
  r : Inport
  Constant : Constant  Value=xdata
  Constant1 : Constant  Value=ydata
  Constant2 : Constant  Value=zdata
  Constant3 : Constant  Value=Tzy_Shard_inv
  Constant4 : Constant  Value=Tzy_Shard
  Constant5 : Constant  Value=u_0
  Constant6 : Constant  Value=u_1
  Constant7 : Constant  Value=u_2
  Demux : Demux  Outputs=3
  MATLAB Function : MATLAB Function  TreatAsAtomicUnit=on
  Matrix Multiply : Product  Multiplication=Matrix(*)
  Matrix Multiply1 : Product  Multiplication=Matrix(*)
  Mux : Mux  Inputs=3
  Out1 : Outport
  wires:
  Demux/1 -> MATLAB Function/7(xpos)
  Demux/2 -> MATLAB Function/8(ypos)
  Demux/3 -> MATLAB Function/9(zpos)
  r/1 -> Matrix Multiply/2  "r^V"
  Constant/1 -> MATLAB Function/4(xdata)
  Constant1/1 -> MATLAB Function/5(ydata)
  Constant2/1 -> MATLAB Function/6(zdata)
  MATLAB Function/1(u0) -> Mux/1
  MATLAB Function/2(u1) -> Mux/2
  Constant3/1 -> Matrix Multiply/1
  Matrix Multiply/1 -> Demux/1
  Constant4/1 -> Matrix Multiply1/1
  Mux/1 -> Matrix Multiply1/2
  Matrix Multiply1/1 -> Out1/1  "v_gust^V"
  MATLAB Function/3(u2) -> Mux/3
  Constant5/1 -> MATLAB Function/1(u_0)
  Constant6/1 -> MATLAB Function/2(u_1)
  Constant7/1 -> MATLAB Function/3(u_2)

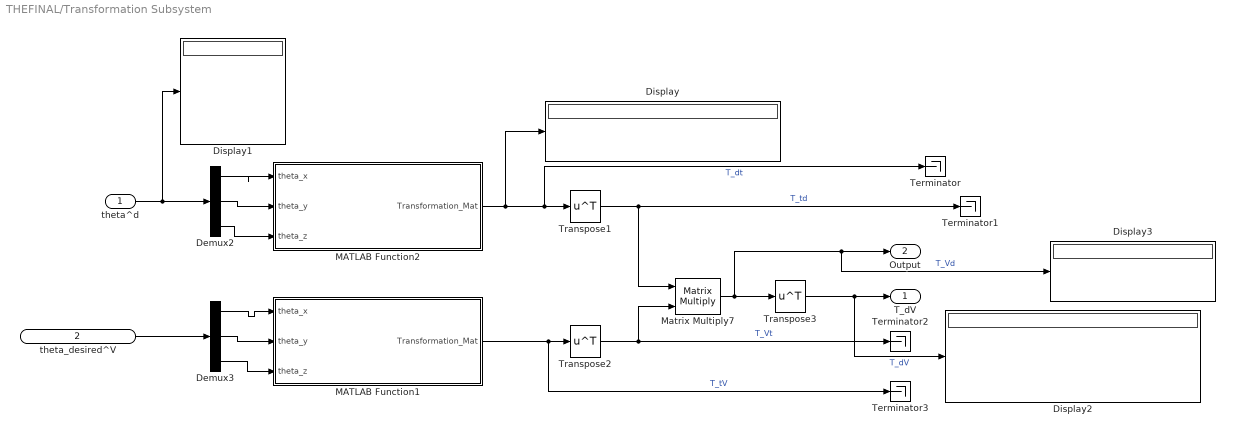
== system THEFINAL/Transformation Subsystem ==
  theta^d : Inport
  theta_desired^V : Inport  Port=2
  Demux2 : Demux  Outputs=3
  Demux3 : Demux  Outputs=3
  Display{,1..3} (4 alike) : Display
  MATLAB Function1 : MATLAB Function  TreatAsAtomicUnit=on
  MATLAB Function2 : MATLAB Function  TreatAsAtomicUnit=on
  Matrix Multiply7 : Product  Multiplication=Matrix(*)
  Terminator{,1..3} (4 alike) : Terminator
  Transpose1 : Math  Operator=transpose  SaturateOnIntegerOverflow=on
  Transpose2 : Math  Operator=transpose  SaturateOnIntegerOverflow=on
  Transpose3 : Math  Operator=transpose  SaturateOnIntegerOverflow=on
  T_dV : Outport
  Output : Outport  Port=2
  wires:
  Demux3/1 -> MATLAB Function1/1(theta_x)
  Demux2/1 -> MATLAB Function2/1(theta_x)
  Transpose2/1 -> Terminator2/1, Matrix Multiply7/2  "T_Vt"
  Demux2/2 -> MATLAB Function2/2(theta_y)
  MATLAB Function2/1(Transformation_Mat) -> Display/1, Terminator/1, Transpose1/1  "T_dt"
  Transpose1/1 -> Terminator1/1, Matrix Multiply7/1  "T_td"
  Demux2/3 -> MATLAB Function2/3(theta_z)
  MATLAB Function1/1(Transformation_Mat) -> Terminator3/1, Transpose2/1  "T_tV"
  Matrix Multiply7/1 -> Display3/1, Output/1, Transpose3/1  "T_Vd"
  theta_desired^V/1 -> Demux3/1
  Demux3/3 -> MATLAB Function1/3(theta_z)
  Demux3/2 -> MATLAB Function1/2(theta_y)
  theta^d/1 -> Display1/1, Demux2/1
  Transpose3/1 -> Display2/1, T_dV/1  "T_dV"

== system THEFINAL/Wind gust1 ==
  Add : Sum  Inputs=+-
  Add1 : Sum  Inputs=+-
  Constant : Constant  Value=12.4
  Constant1 : Constant  Value=4.25
  Constant2 : Constant
  Constant3 : Constant  Value=0
  Constant4 : Constant  Value=0  VectorParams1D=off
  Mux : Mux  Inputs=3
  Product : Product
  Product1 : Product
  Sine Wave : Sin  Frequency=3*pi/T  SampleTime=0
  Sine Wave1 : Sin  Frequency=2*pi/T  Phase=pi/2  SampleTime=0
  V_tot : Outport
  wires:
  Constant/1 -> Add/1
  Constant1/1 -> Product/1
  Sine Wave/1 -> Product/2
  Constant2/1 -> Add1/1
  Sine Wave1/1 -> Add1/2
  Product/1 -> Product1/1
  Add1/1 -> Product1/2
  Product1/1 -> Add/2
  Add/1 -> Mux/2  "v_gust_y"
  Constant3/1 -> Mux/3  "v_gust_z"
  Constant4/1 -> Mux/1  "v_gust_x"
  Mux/1 -> V_tot/1

== system THEFINAL/Propulsion commands module/Propeller firing function ==
  Fc(t-tau) : Inport
  T_dV : Inport  Port=2
  M_control_d : Inport  Port=3
  Gain6 : Gain
  MATLAB Function : MATLAB Function  TreatAsAtomicUnit=on
  Matrix Multiply5 : Product  Multiplication=Matrix(*)
  To Workspace : ToWorkspace  VariableName=Fc_wanted  SaveFormat=Timeseries  SampleTime=-1
  To Workspace1 : ToWorkspace  VariableName=Ft_wanted  SaveFormat=Timeseries  SampleTime=-1
  To Workspace2 : ToWorkspace  VariableName=Fb_wanted  SaveFormat=Timeseries  SampleTime=-1
  Turn off for PID tune : Gain
  Output : Outport
  Output1 : Outport  Port=2
  Output2 : Outport  Port=3
  wires:
  Turn off for PID tune/1 -> Matrix Multiply5/2
  Fc(t-tau)/1 -> Turn off for PID tune/1
  Matrix Multiply5/1 -> MATLAB Function/1(F_wanted)  "F_c_d"
  M_control_d/1 -> Gain6/1
  Gain6/1 -> MATLAB Function/2(M_wanted)  "M_c_d"
  MATLAB Function/2(F_t) -> To Workspace1/1, Output1/1  "Ft_wanted"
  MATLAB Function/3(F_b) -> Output2/1, To Workspace2/1  "Fb_wanted"
  MATLAB Function/1(F_c) -> To Workspace/1, Output/1  "Fc_wanted"
  T_dV/1 -> Matrix Multiply5/1

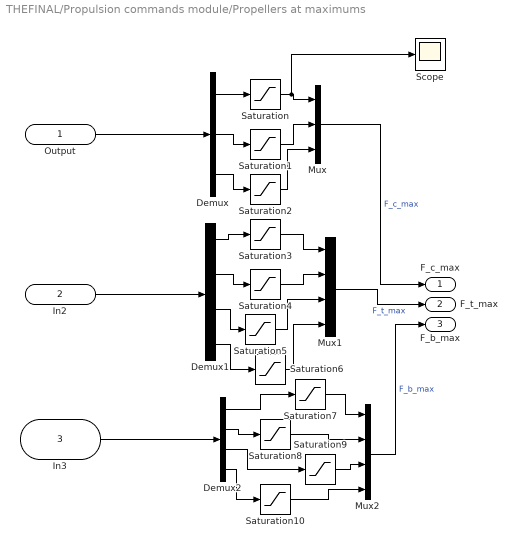
== system THEFINAL/Propulsion commands module/Propellers at maximums ==
  Output : Inport
  In2 : Inport  Port=2
  In3 : Inport  Port=3
  Demux : Demux  Outputs=3
  Demux1 : Demux
  Demux2 : Demux
  Mux : Mux  Inputs=3
  Mux1 : Mux
  Mux2 : Mux
  Saturation : Saturate  UpperLimit=Fc1_u  LowerLimit=Fc1_l
  Saturation1 : Saturate  UpperLimit=Fc2_u  LowerLimit=Fc2_l
  Saturation10 : Saturate  UpperLimit=Fb4_u  LowerLimit=Fb4_l
  Saturation2 : Saturate  UpperLimit=Fc3_u  LowerLimit=Fc3_l
  Saturation3 : Saturate  UpperLimit=Ft1_u  LowerLimit=Ft1_l
  Saturation4 : Saturate  UpperLimit=Ft2_u  LowerLimit=Ft2_l
  Saturation5 : Saturate  UpperLimit=Ft3_u  LowerLimit=Ft3_l
  Saturation6 : Saturate  UpperLimit=Ft4_u  LowerLimit=Ft4_l
  Saturation7 : Saturate  UpperLimit=Fb1_u  LowerLimit=Fb1_l
  Saturation8 : Saturate  UpperLimit=Fb2_u  LowerLimit=Fb2_l
  Saturation9 : Saturate  UpperLimit=Fb3_u  LowerLimit=Fb3_l
  Scope : Scope
  F_c_max : Outport
  F_t_max : Outport  Port=2
  F_b_max : Outport  Port=3
  wires:
  Demux2/1 -> Saturation7/1
  Output/1 -> Demux/1
  Saturation2/1 -> Mux/3
  Mux2/1 -> F_b_max/1  "F_b_max"
  Demux2/2 -> Saturation8/1
  Demux/1 -> Saturation/1
  Demux/2 -> Saturation1/1
  Demux2/3 -> Saturation9/1
  Demux1/1 -> Saturation3/1
  Saturation3/1 -> Mux1/1
  Saturation7/1 -> Mux2/1
  Demux1/4 -> Saturation6/1
  Demux2/4 -> Saturation10/1
  Saturation6/1 -> Mux1/4
  Mux/1 -> F_c_max/1  "F_c_max"
  Saturation/1 -> Scope/1, Mux/1
  Saturation1/1 -> Mux/2
  Mux1/1 -> F_t_max/1  "F_t_max"
  Saturation5/1 -> Mux1/3
  Demux/3 -> Saturation2/1
  Saturation4/1 -> Mux1/2
  Demux1/2 -> Saturation4/1
  Demux1/3 -> Saturation5/1
  Saturation8/1 -> Mux2/2
  Saturation9/1 -> Mux2/3
  Saturation10/1 -> Mux2/4
  In3/1 -> Demux2/1
  In2/1 -> Demux1/1

== system THEFINAL/Propulsion commands module/Subsystem3 ==
  Fc : Inport
  Ft : Inport  Port=2
  Fb : Inport  Port=3
  MATLAB Function : MATLAB Function  TreatAsAtomicUnit=on
  Fx_acc : Outport
  Fy_acc : Outport  Port=2
  Fz_acc : Outport  Port=3
  Mx_acc : Outport  Port=4
  My_acc : Outport  Port=5
  Mz_acc : Outport  Port=6
  wires:
  Fc/1 -> MATLAB Function/1(Fc)
  Ft/1 -> MATLAB Function/2(Ft)
  Fb/1 -> MATLAB Function/3(Fb)
  MATLAB Function/1(Fx_acc) -> Fx_acc/1
  MATLAB Function/2(Fy_acc) -> Fy_acc/1
  MATLAB Function/3(Fz_acc) -> Fz_acc/1
  MATLAB Function/4(Mx_acc) -> Mx_acc/1
  MATLAB Function/5(My_acc) -> My_acc/1
  MATLAB Function/6(Mz_acc) -> Mz_acc/1

== system THEFINAL/Propulsion commands module/Subsystem4 ==
  In1 : Inport
  Fy_actual : Inport  Port=2
  Fz_actual : Inport  Port=3
  In4 : Inport  Port=4
  In5 : Inport  Port=5
  In6 : Inport  Port=6
  T_Vd : Inport  Port=7
  Matrix Multiply : Product  Multiplication=Matrix(*)
  Mux : Mux  Inputs=3
  Mux1 : Mux  Inputs=3
  F_c : Outport
  y : Outport  Port=2
  wires:
  In1/1 -> Mux/1
  Fy_actual/1 -> Mux/2
  Fz_actual/1 -> Mux/3
  Matrix Multiply/1 -> F_c/1  "Fc(t-tau)_actual"
  Mux/1 -> Matrix Multiply/2
  Mux1/1 -> y/1  "Mc(t-tau)_actual"
  In4/1 -> Mux1/1  "M_x_acc"
  In5/1 -> Mux1/2  "M_y_acc"
  In6/1 -> Mux1/3  "M_z_acc"
  T_Vd/1 -> Matrix Multiply/1

== system THEFINAL/Propulsion commands module/Top and Bottom including weight counteraction ==
  F_b : Inport
  In2 : Inport  Port=2
  Add : Sum
  Add1 : Sum
  Constant : Constant  Value=m*g
  Gain : Gain  Gain=1/8
  Mux : Mux
  Scope : Scope
  To Workspace : ToWorkspace  VariableName=Ft_inclift  SaveFormat=Timeseries  SampleTime=-1
  To Workspace1 : ToWorkspace  VariableName=Fb_inclift  SaveFormat=Timeseries  SampleTime=-1
  wires:
  Constant/1 -> Mux/4, Mux/3, Mux/2, Mux/1
  Add1/1 -> To Workspace1/1
  F_b/1 -> Add1/1  "F_b"
  In2/1 -> Add/1  "F_t"
  Add/1 -> Scope/1, To Workspace/1
  Gain/1 -> Add1/2, Add/2
  Mux/1 -> Gain/1

== system THEFINAL/Subsystem/Drag1 ==
  note: Change to C_D and S per side
  In1 : Inport
  Constant1 : Constant  Value=2
  Constant4 : Constant  Value=0.5*rho*C_D*S
  Demux : Demux  Outputs=3
  Gain : Gain  Gain=0
  Mux : Mux  Inputs=3
  Power : Math  Operator=pow  SaturateOnIntegerOverflow=on
  Power1 : Math  Operator=pow  SaturateOnIntegerOverflow=on
  Power2 : Math  Operator=pow  SaturateOnIntegerOverflow=on
  Product1 : Product
  Out1 : Outport
  drag : Outport  Port=2
  wires:
  Constant1/1 -> Power2/2, Power1/2, Power/2
  Power2/1 -> Mux/3
  Power/1 -> Gain/1
  In1/1 -> Demux/1
  Demux/1 -> Power/1
  Demux/3 -> Power2/1
  Demux/2 -> Power1/1
  Power1/1 -> Mux/2
  Constant4/1 -> Product1/2
  Mux/1 -> Out1/1, Product1/1
  Product1/1 -> drag/1  "drag"
  Gain/1 -> Mux/1

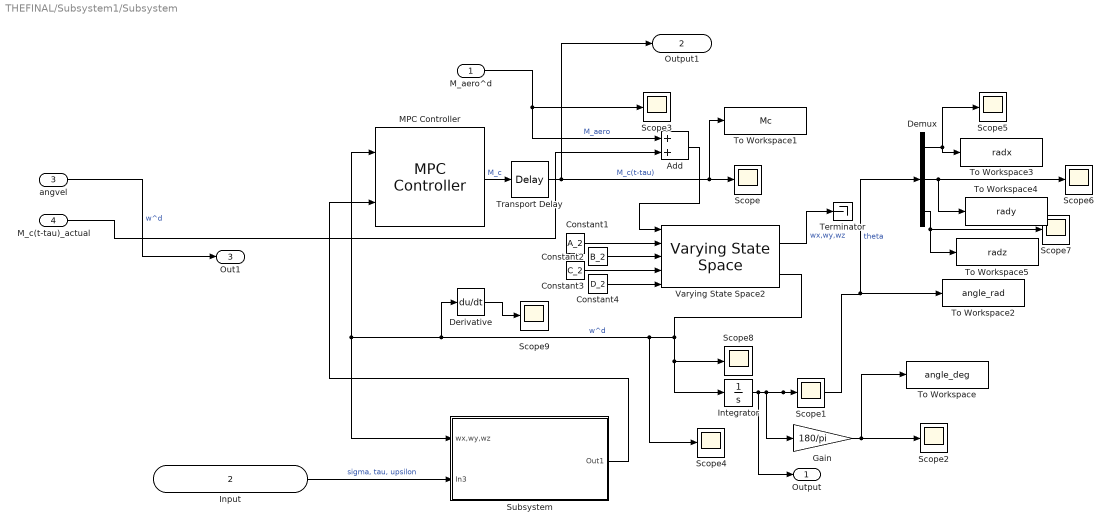
== system THEFINAL/Subsystem1/Subsystem ==
  M_aero^d : Inport
  Input : Inport  Port=2
  angvel : Inport  Port=3
  M_c(t-tau)_actual : Inport  Port=4
  Add : Sum
  Constant1 : Constant  Value=A_2
  Constant2 : Constant  Value=B_2
  Constant3 : Constant  Value=C_2
  Constant4 : Constant  Value=D_2
  Demux : Demux  Outputs=3
  Derivative : Derivative
  Gain : Gain  Gain=180/pi
  Integrator : Integrator
  MPC Controller : mpclib/MPC Controller  SCDEnableBlockLinearizationSpecification=on  mpcobj=MPCDesignerSession.AppData.Controllers.MPC  is_multiple=0  enable_value=0  return_u0=off  updateMPCinCallerWorkspace=on  md_inport=off  mv_inport=off  uref_inport=off  return_cost=off  return_mvseq=off  return_qpstatus=off  return_xseq=off  return_state=off  return_ovseq=off  state_inport=off  umin_inport=off  umax_inport=off  ymin_inport=off  ymax_inport=off  cc_inport=off  ywt_inport=off  uwt_inport=off  duwt_inport=off  rhoeps_inport=off  pm_inport=off  MaximumP=10  HorizonChoice=FixedHorizon  n_ts=0.1  n_p=10  n_mv=3  n_md=0  n_ud=0  n_mo=3  n_uo=0  BlockDataType=double  SampleTimeInherited=off  switch_inport=off
  Scope{,1..9} (10 alike) : Scope
  Subsystem : Subsystem
  Terminator : Terminator
  To Workspace : ToWorkspace  VariableName=angle_deg  SaveFormat=Timeseries  SampleTime=-1
  To Workspace1 : ToWorkspace  VariableName=Mc  SaveFormat=Timeseries  SampleTime=-1
      settings: Save2DSignal=2-D array (concatenate along first dimension)
  To Workspace2 : ToWorkspace  VariableName=angle_rad  SaveFormat=Timeseries  SampleTime=-1
  To Workspace3 : ToWorkspace  VariableName=radx  SaveFormat=Timeseries  SampleTime=-1
  To Workspace4 : ToWorkspace  VariableName=rady  SaveFormat=Timeseries  SampleTime=-1
  To Workspace5 : ToWorkspace  VariableName=radz  SaveFormat=Timeseries  SampleTime=-1
  Transport Delay : TransportDelay  DelayTime=0.1
  Varying State Space2 : cstblocks/Linear Parameter Varying/Varying State Space  x0=0  xNames=''  OutputX=on  OutputDX=off
  Output : Outport
  Output1 : Outport  Port=2
  Out1 : Outport  Port=3
  wires:
  Demux/3 -> To Workspace5/1, Scope7/1
  Subsystem/1(Out1) -> MPC Controller/2
  Constant1/1 -> Varying State Space2/2
  MPC Controller/1 -> Transport Delay/1  "M_c"
  Derivative/1 -> Scope9/1
  Demux/1 -> Scope5/1, To Workspace3/1
  Constant4/1 -> Varying State Space2/5
  Demux/2 -> To Workspace4/1, Scope6/1
  Gain/1 -> To Workspace/1, Scope2/1
  Integrator/1 -> Demux/1, To Workspace2/1, Scope1/1, Gain/1, Output/1  "theta"
  Input/1 -> Subsystem/2(In3)  "sigma, tau, upsilon"
  Add/1 -> Varying State Space2/1
  Varying State Space2/1 -> Terminator/1  "wx,wy,wz"
  Constant2/1 -> Varying State Space2/3
  Constant3/1 -> Varying State Space2/4
  Transport Delay/1 -> Output1/1, To Workspace1/1, Scope/1  "M_c(t-tau)"
  M_aero^d/1 -> Scope3/1, Add/1  "M_aero"
  Varying State Space2/2 -> Scope8/1, Integrator/1, MPC Controller/1, Subsystem/1(wx,wy,wz), Derivative/1, Scope4/1  "w^d"
  angvel/1 -> Out1/1  "w^d"
  M_c(t-tau)_actual/1 -> Add/2

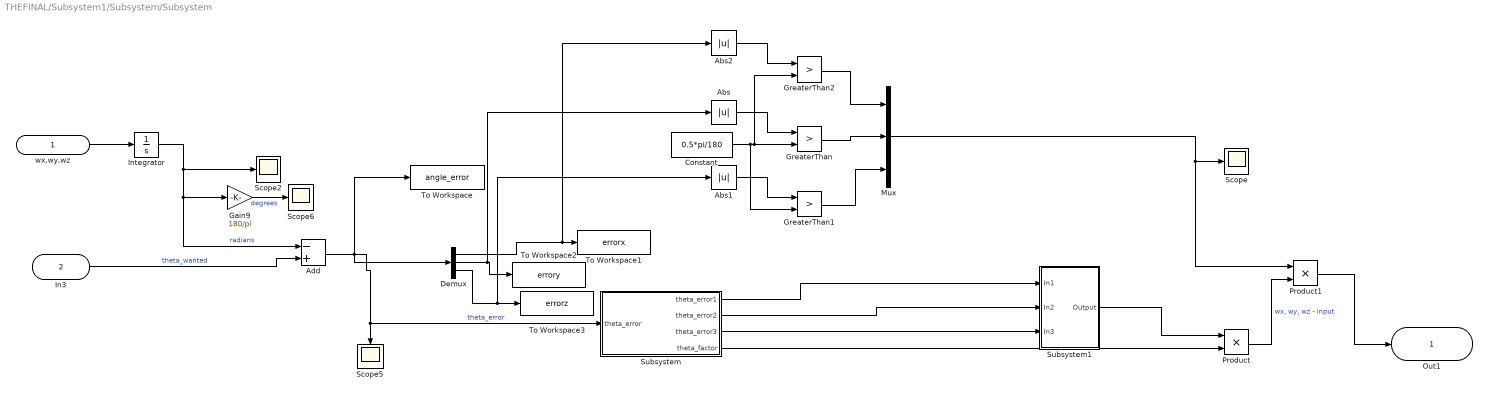
== system THEFINAL/Subsystem1/Subsystem/Subsystem ==
  wx,wy,wz : Inport
  In3 : Inport  Port=2
  Abs : Abs
  Abs1 : Abs
  Abs2 : Abs
  Add : Sum  Inputs=-+
  Constant : Constant  Value=0.5*pi/180
  Demux : Demux  Outputs=3
  Gain9 : Gain  Gain=180/pi
  GreaterThan : RelationalOperator  Operator=>  OutDataTypeStr=boolean  RndMeth=Simplest
  GreaterThan1 : RelationalOperator  Operator=>  OutDataTypeStr=boolean  RndMeth=Simplest
  GreaterThan2 : RelationalOperator  Operator=>  OutDataTypeStr=boolean  RndMeth=Simplest
  Integrator : Integrator
  Mux : Mux  Inputs=3
  Product : Product
  Product1 : Product
  Scope{,2,5..6} (4 alike) : Scope
  Subsystem : Subsystem
  Subsystem1 : Subsystem
  To Workspace : ToWorkspace  VariableName=angle_error  SampleTime=-1
  To Workspace1 : ToWorkspace  VariableName=errorx  SaveFormat=Timeseries  SampleTime=-1
      settings: Save2DSignal=2-D array (concatenate along first dimension)
  To Workspace2 : ToWorkspace  VariableName=errory  SaveFormat=Timeseries  SampleTime=-1
  To Workspace3 : ToWorkspace  VariableName=errorz  SaveFormat=Timeseries  SampleTime=-1
  Out1 : Outport
  wires:
  Integrator/1 -> Add/1, Gain9/1, Scope2/1  "radians"
  Add/1 -> To Workspace/1, Demux/1, Subsystem/1(theta_error), Scope5/1  "theta_error"
  Gain9/1 -> Scope6/1  "degrees"
  In3/1 -> Add/2  "theta_wanted"
  Product/1 -> Product1/2  "wx, wy, wz - input"
  wx,wy,wz/1 -> Integrator/1
  Subsystem/4(theta_factor) -> Product/2
  Demux/2 -> Abs/1, To Workspace2/1
  Demux/3 -> Abs1/1, To Workspace3/1
  Demux/1 -> Abs2/1, To Workspace1/1
  Subsystem/1(theta_error1) -> Subsystem1/1(In1)
  Subsystem/2(theta_error2) -> Subsystem1/2(In2)
  Subsystem/3(theta_error3) -> Subsystem1/3(In3)
  Subsystem1/1(Output) -> Product/1
  Abs/1 -> GreaterThan/1
  Constant/1 -> GreaterThan1/2, GreaterThan2/2, GreaterThan/2
  Abs1/1 -> GreaterThan1/1
  Abs2/1 -> GreaterThan2/1
  GreaterThan2/1 -> Mux/1
  GreaterThan/1 -> Mux/2
  GreaterThan1/1 -> Mux/3
  Mux/1 -> Scope/1, Product1/1
  Product1/1 -> Out1/1
